simulink model "Direct_Form_Test_Model"  (R2019b)
settings: Solver=VariableStepAuto  StartTime=0.0  StopTime=testtime  RelTol=1e-3
InitFcn:
  | Direct_Form_Test_Parameters
StopFcn:
  | Verify_Direct_Form_Filter
undefined symbols (not defined in the file or in its folder): Fs, INCLPcoeffs
libraries: dspsrcs4 x1
settings Model: Creator=mblun  LastModifiedBy=cb50701
settings OptimizationCC: BlockReduction=off  ConditionallyExecuteInputs=off  DefaultParameterBehavior=Inlined
settings DebuggingCC: AlgebraicLoopMsg=error
settings HardwareCC: ProdBitPerPointer=32  ProdBitPerSizeT=32  ProdBitPerPtrDiffT=32  ProdLargestAtomicFloat=None  ProdIntDivRoundTo=Undefined  ProdEndianess=Unspecified  ProdWordSize=32  ProdHWDeviceType=ASIC/FPGA->ASIC/FPGA  TargetBitPerLong=64  TargetBitPerPointer=64  TargetBitPerSizeT=64  TargetBitPerPtrDiffT=64  TargetLongLongMode=on  TargetIntDivRoundTo=Zero  TargetEndianess=LittleEndian  TargetWordSize=64  TargetHWDeviceType=Custom Processor->MATLAB Host Computer  ProdEqTarget=off
settings SFSimCC: CustomCodeUndefinedFunction=UseInterfaceOnly

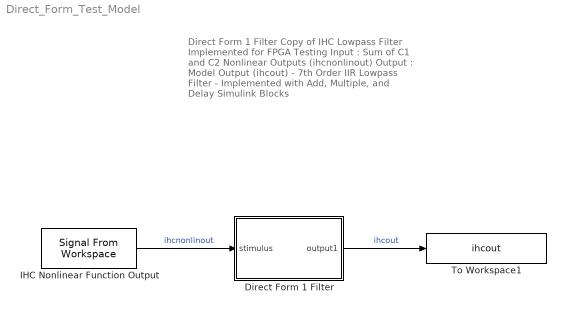
== system Direct_Form_Test_Model ==
  note: Direct Form 1 Filter
      | Copy of IHC Lowpass Filter
      | Implemented for FPGA Testing
      |
      | Input : Sum of C1 and C2 Nonlinear Outputs (ihcnonlinout)
      |
      | Output : Model Output (ihcout)
      |
      | - 7th Order IIR Lowpass Filter
      |
      | - Implemented with Add, Multiple, and Delay Simulink Blocks
  Direct Form 1 Filter : Subsystem
  IHC Nonlinear Function Output : dspsrcs4/Signal From Workspace  X=RxSignal  Ts=1/Fs  nsamps=1  OutputAfterFinalValue=Setting to zero  ignoreOrWarnInputAndFrameLengths=off  OutputFrames=off
  To Workspace1 : ToWorkspace  VariableName=ihcout  SampleTime=-1
      settings: Save2DSignal=2-D array (concatenate along first dimension)
  wires:
  IHC Nonlinear Function Output/1 -> Direct Form 1 Filter/1(stimulus)  "ihcnonlinout"
  Direct Form 1 Filter/1(output1) -> To Workspace1/1  "ihcout"

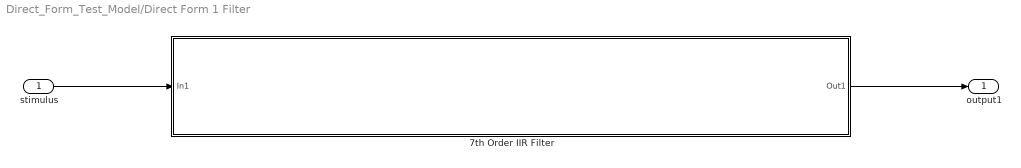
== system Direct_Form_Test_Model/Direct Form 1 Filter ==
  stimulus : Inport
  7th Order IIR Filter : Subsystem
  output1 : Outport  VectorParamsAs1DForOutWhenUnconnected=off
  wires:
  stimulus/1 -> 7th Order IIR Filter/1(In1)
  7th Order IIR Filter/1(Out1) -> output1/1

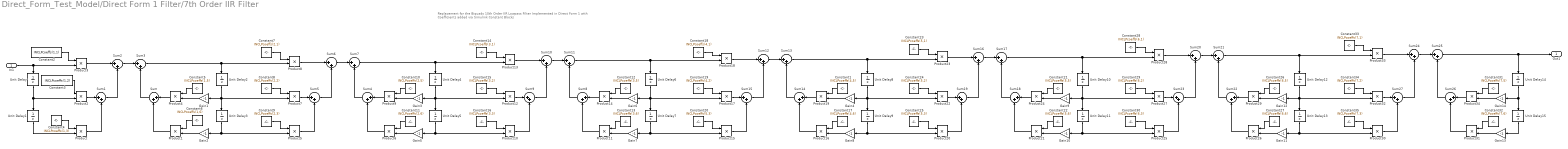
== system Direct_Form_Test_Model/Direct Form 1 Filter/7th Order IIR Filter ==
  note: Replacement for the Biquads
      | 10th Order IIR Lowpass Filter Implemented in Direct Form 1 with Coefficients added via Simulink Constant Blocks
  In1 : Inport  OutDataTypeStr=single
  Constant1 : Constant  Value=INCLPcoeffs(4,5)  OutDataTypeStr=single  SampleTime=-1
  Constant10 : Constant  Value=INCLPcoeffs(2,5)  OutDataTypeStr=single  SampleTime=-1
  Constant11 : Constant  Value=INCLPcoeffs(2,6)  OutDataTypeStr=single  SampleTime=-1
  Constant12 : Constant  Value=INCLPcoeffs(3,5)  OutDataTypeStr=single  SampleTime=-1
  Constant13 : Constant  Value=INCLPcoeffs(3,6)  OutDataTypeStr=single  SampleTime=-1
  Constant14 : Constant  Value=INCLPcoeffs(3,1)  OutDataTypeStr=single  SampleTime=-1
  Constant15 : Constant  Value=INCLPcoeffs(3,2)  OutDataTypeStr=single  SampleTime=-1
  Constant16 : Constant  Value=INCLPcoeffs(3,3)  OutDataTypeStr=single  SampleTime=-1
  Constant17 : Constant  Value=INCLPcoeffs(4,6)  OutDataTypeStr=single  SampleTime=-1
  Constant18 : Constant  Value=INCLPcoeffs(4,1)  OutDataTypeStr=single  SampleTime=-1
  Constant19 : Constant  Value=INCLPcoeffs(4,2)  OutDataTypeStr=single  SampleTime=-1
  Constant2 : Constant  Value=INCLPcoeffs(1,1)  OutDataTypeStr=single  SampleTime=-1
  Constant20 : Constant  Value=INCLPcoeffs(5,3)  OutDataTypeStr=single  SampleTime=-1
  Constant21 : Constant  Value=INCLPcoeffs(5,5)  OutDataTypeStr=single  SampleTime=-1
  Constant22 : Constant  Value=INCLPcoeffs(5,6)  OutDataTypeStr=single  SampleTime=-1
  Constant23 : Constant  Value=INCLPcoeffs(5,1)  OutDataTypeStr=single  SampleTime=-1
  Constant24 : Constant  Value=INCLPcoeffs(5,2)  OutDataTypeStr=single  SampleTime=-1
  Constant25 : Constant  Value=INCLPcoeffs(5,3)  OutDataTypeStr=single  SampleTime=-1
  Constant26 : Constant  Value=INCLPcoeffs(6,5)  OutDataTypeStr=single  SampleTime=-1
  Constant27 : Constant  Value=INCLPcoeffs(6,6)  OutDataTypeStr=single  SampleTime=-1
  Constant28 : Constant  Value=INCLPcoeffs(6,1)  OutDataTypeStr=single  SampleTime=-1
  Constant29 : Constant  Value=INCLPcoeffs(6,2)  OutDataTypeStr=single  SampleTime=-1
  Constant3 : Constant  Value=INCLPcoeffs(1,2)  OutDataTypeStr=single  SampleTime=-1
  Constant30 : Constant  Value=INCLPcoeffs(6,3)  OutDataTypeStr=single  SampleTime=-1
  Constant31 : Constant  Value=INCLPcoeffs(7,5)  OutDataTypeStr=single  SampleTime=-1
  Constant32 : Constant  Value=INCLPcoeffs(7,6)  OutDataTypeStr=single  SampleTime=-1
  Constant33 : Constant  Value=INCLPcoeffs(7,1)  OutDataTypeStr=single  SampleTime=-1
  Constant34 : Constant  Value=INCLPcoeffs(7,2)  OutDataTypeStr=single  SampleTime=-1
  Constant35 : Constant  Value=INCLPcoeffs(7,3)  OutDataTypeStr=single  SampleTime=-1
  Constant4 : Constant  Value=INCLPcoeffs(1,3)  OutDataTypeStr=single  SampleTime=-1
  Constant5 : Constant  Value=INCLPcoeffs(1,5)  OutDataTypeStr=single  SampleTime=-1
  Constant6 : Constant  Value=INCLPcoeffs(1,6)  OutDataTypeStr=single  SampleTime=-1
  Constant7 : Constant  Value=INCLPcoeffs(2,1)  OutDataTypeStr=single  SampleTime=-1
  Constant8 : Constant  Value=INCLPcoeffs(2,2)  OutDataTypeStr=single  SampleTime=-1
  Constant9 : Constant  Value=INCLPcoeffs(2,3)  OutDataTypeStr=single  SampleTime=-1
  Gain{1..14} (14 alike) : Gain  Gain=-1
  Product{,1..34} (35 alike) : Product
  Sum{,1..27} (28 alike) : Sum  Inputs=|++
  Unit Delay{,1..15} (16 alike) : UnitDelay  SampleTime=-1  HasFrameUpgradeWarning=on
  Out1 : Outport  OutDataTypeStr=single
  wires:
  Sum5/1 -> Sum6/2
  Product/1 -> Sum1/2
  Constant6/1 -> Product1/1
  Sum1/1 -> Sum2/2
  Sum6/1 -> Sum7/1
  Sum2/1 -> Sum3/1
  Constant8/1 -> Product7/1
  Sum14/1 -> Sum13/2
  Constant10/1 -> Product9/1
  Product5/1 -> Sum5/2
  Product2/1 -> Sum1/1
  Gain10/1 -> Product21/2
  Constant5/1 -> Product4/1
  Unit Delay11/1 -> Product25/2, Gain10/1
  Constant4/1 -> Product/1
  Sum4/1 -> Sum7/2
  Constant18/1 -> Product18/1
  Constant12/1 -> Product14/1
  Product4/1 -> Sum/1
  Product17/1 -> Sum15/1
  Constant14/1 -> Product13/1
  Gain2/1 -> Product1/2
  Sum17/1 -> Unit Delay10/1, Product28/2
  Product13/1 -> Sum10/1
  Sum15/1 -> Sum12/2
  Product10/1 -> Sum9/2
  Gain3/1 -> Product9/2
  Unit Delay/1 -> Unit Delay1/1, Product2/2
  Unit Delay8/1 -> Product22/2, Unit Delay9/1, Gain4/1
  Sum19/1 -> Sum16/2
  Constant16/1 -> Product10/1
  Product9/1 -> Sum4/1
  Sum3/1 -> Unit Delay2/1, Product8/2
  Product23/1 -> Sum16/1
  Product3/1 -> Sum2/1
  Product20/1 -> Sum19/2
  Constant3/1 -> Product2/1
  Constant21/1 -> Product24/1
  Unit Delay2/1 -> Product7/2, Unit Delay3/1, Gain1/1
  Unit Delay7/1 -> Product15/2, Gain7/1
  Constant19/1 -> Product17/1
  Constant9/1 -> Product5/1
  Sum16/1 -> Sum17/1
  Constant22/1 -> Product21/1
  Constant15/1 -> Product12/1
  Product18/1 -> Sum12/1
  Constant13/1 -> Product11/1
  Sum11/1 -> Unit Delay6/1, Product18/2
  Sum/1 -> Sum3/2
  Unit Delay6/1 -> Product17/2, Unit Delay7/1, Gain6/1
  Unit Delay10/1 -> Product27/2, Unit Delay11/1, Gain9/1
  Gain9/1 -> Product24/2
  Gain5/1 -> Product6/2
  Product14/1 -> Sum8/1
  Sum10/1 -> Sum11/1
  Gain4/1 -> Product19/2
  Sum8/1 -> Sum11/2
  Constant17/1 -> Product16/1
  Gain1/1 -> Product4/2
  Sum9/1 -> Sum10/2
  Gain7/1 -> Product11/2
  Product6/1 -> Sum4/2
  Unit Delay1/1 -> Product/2
  Sum7/1 -> Unit Delay4/1, Product13/2
  Constant11/1 -> Product6/1
  Constant25/1 -> Product20/1
  Sum13/1 -> Unit Delay8/1, Product23/2
  Unit Delay5/1 -> Product10/2, Gain5/1
  Product16/1 -> Sum14/2
  Gain6/1 -> Product14/2
  Product7/1 -> Sum5/1
  Product22/1 -> Sum19/1
  Product15/1 -> Sum15/2
  Unit Delay3/1 -> Product5/2, Gain2/1
  Product11/1 -> Sum8/2
  Constant24/1 -> Product22/1
  Sum18/1 -> Sum17/2
  Constant20/1 -> Product15/1
  Product12/1 -> Sum9/1
  Unit Delay9/1 -> Product20/2, Gain8/1
  Unit Delay4/1 -> Product12/2, Unit Delay5/1, Gain3/1
  Constant1/1 -> Product19/1
  Product8/1 -> Sum6/1
  Gain8/1 -> Product16/2
  In1/1 -> Product3/2, Unit Delay/1
  Constant7/1 -> Product8/1
  Constant2/1 -> Product3/1
  Product21/1 -> Sum18/2
  Constant23/1 -> Product23/1
  Product24/1 -> Sum18/1
  Product1/1 -> Sum/2
  Product19/1 -> Sum14/1
  Sum12/1 -> Sum13/1
  Constant28/1 -> Product28/1
  Product26/1 -> Sum22/2
  Constant29/1 -> Product27/1
  Unit Delay12/1 -> Product32/2, Unit Delay13/1, Gain12/1
  Product28/1 -> Sum20/1
  Product27/1 -> Sum23/1
  Sum23/1 -> Sum20/2
  Gain11/1 -> Product26/2
  Sum21/1 -> Unit Delay12/1, Product33/2
  Gain12/1 -> Product29/2
  Unit Delay13/1 -> Product30/2, Gain11/1
  Product25/1 -> Sum23/2
  Sum20/1 -> Sum21/1
  Constant30/1 -> Product25/1
  Constant27/1 -> Product26/1
  Sum22/1 -> Sum21/2
  Constant26/1 -> Product29/1
  Product29/1 -> Sum22/1
  Constant33/1 -> Product33/1
  Product31/1 -> Sum26/2
  Constant34/1 -> Product32/1
  Unit Delay14/1 -> Unit Delay15/1, Gain14/1
  Product33/1 -> Sum24/1
  Product32/1 -> Sum27/1
  Sum27/1 -> Sum24/2
  Gain13/1 -> Product31/2
  Sum25/1 -> Out1/1, Unit Delay14/1
  Gain14/1 -> Product34/2
  Unit Delay15/1 -> Gain13/1
  Product30/1 -> Sum27/2
  Sum24/1 -> Sum25/1
  Constant35/1 -> Product30/1
  Constant32/1 -> Product31/1
  Sum26/1 -> Sum25/2
  Constant31/1 -> Product34/1
  Product34/1 -> Sum26/1
